simulink model "EKF_sim"  (R2021a)
settings: Solver=ode45  StartTime=0.0  StopTime=450  MaxStep=0.1  RelTol=1e-3  EnableMultiTasking=on
model workspace (MATLAB code in the model file + MAT data in the model file):
  L = 2.5
  v0 = 0
  xe0 = 0
  xn0 = 0
  theta0 = 0
  Ts = 1
  rr = [0 0 0 0 0 0 0 0 0 0 0 0 ... (9404 elements, 9404x1)]
  tt = [0 0.05 0.1 0.15 0.2 0.25 0.3 0.35 0.4 0.45 0.5 0.55 ... (9404 elements, 9404x1)]
  vv = [25 25 25 25 25 25 25 25 25 25 25 25 ... (9404 elements, 9404x1)]
libraries: simulink x2, pid_lib x2, sharedTrackingLibrary x1
(part 1 of 2)
settings Model: Creator=The MathWorks, Inc.  LastModifiedBy=angeloz
settings SolverCC: AlgebraicLoopSolver=TrustRegion
settings DataIOCC: SaveFormat=Array  SaveOutput=off  SignalLogging=off  DSMLogging=off  SaveTime=off  ReturnWorkspaceOutputs=off
settings OptimizationCC: LifeSpan=inf
settings DebuggingCC: AlgebraicLoopMsg=none  SolverPrmCheckMsg=warning  SFUnexpectedBacktrackingDiag=warning  SFNoUnconditionalDefaultTransitionDiag=warning  SFExecutionAtInitializationDiag=none  SFMachineParentedDataDiag=warning  ArithmeticOperatorsInVariantConditions=warning
settings HardwareCC: ProdBitPerPointer=32  ProdBitPerSizeT=32  ProdBitPerPtrDiffT=32  ProdLargestAtomicFloat=None  ProdIntDivRoundTo=Undefined  ProdEndianess=Unspecified  ProdWordSize=32  ProdHWDeviceType=32-bit Generic
settings ModelReferenceCC: PropagateSignalLabelsOutOfModel=off
settings SFSimCC: SimUseLocalCustomCode=off  CustomCodeUndefinedFunction=UseInterfaceOnly
settings RTWCC: RTWUseLocalCustomCode=off
settings CodeAppCC: StateflowObjectComments=on
settings GRTTargetCC: TargetLangStandard=C89/C90 (ANSI)
settings ConfigComp: CovMetricSettings=dw  CovSaveCumulativeToWorkspaceVar=on  CovSaveSingleToWorkspaceVar=on  CovExternalEMLEnable=off  CovSFcnEnable=off

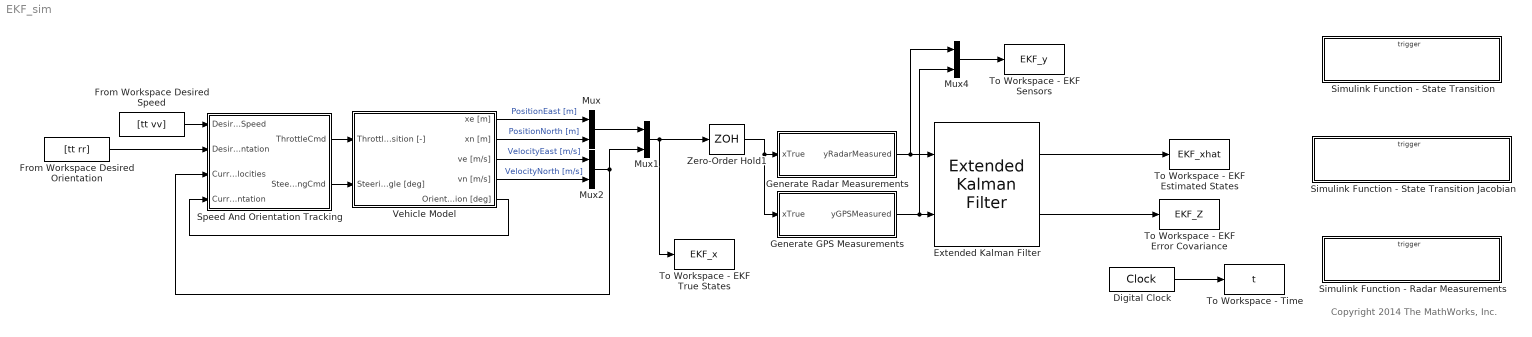
== system EKF_sim ==
  note: Copyright 2014 The MathWorks, Inc.
  Digital Clock : DigitalClock  SampleTime=Ts
  Extended Kalman Filter : sharedTrackingLibrary/Extended Kalman Filter  StateTransitionFcn=stateTransitionFcn  HasStateTransitionJacobianFcn=on  StateTransitionJacobianFcn=stateTransitionJacobianFcn  HasAdditiveProcessNoise=Nonadditive  ProcessNoise=[0.01 0; 0 0.01]  HasTimeVaryingProcessNoise=off  HasStateTransitionFcnExtraArgument=0  InitialState=[0; 0; 0; 0]  InitialStateCovariance=10  MeasurementFcn1=radarMeasurementFcn  HasMeasurementJacobianFcn1=off  HasMeasurementEnablePort1=off  HasAdditiveMeasurementNoise1=Nonadditive  MeasurementNoise1=[0.0025 0; 0 0.0025]  HasTimeVaryingMeasurementNoise1=off  HasMeasurementFcnExtraArgument1=0  MeasurementFcn2=gpsMeasurementFcn  HasMeasurementJacobianFcn2=off  HasMeasurementEnablePort2=off  HasAdditiveMeasurementNoise2=Additive  MeasurementNoise2=[100 0; 0 100]  HasTimeVaryingMeasurementNoise2=off  HasMeasurementFcnExtraArgument2=0  MeasurementFcn3=myMeasurementFcn  HasMeasurementJacobianFcn3=off  HasMeasurementEnablePort3=off  HasAdditiveMeasurementNoise3=Additive  MeasurementNoise3=1  HasTimeVaryingMeasurementNoise3=off  HasMeasurementFcnExtraArgument3=0  MeasurementFcn4=myMeasurementFcn  HasMeasurementJacobianFcn4=off  HasMeasurementEnablePort4=off  HasAdditiveMeasurementNoise4=Additive  MeasurementNoise4=1  HasTimeVaryingMeasurementNoise4=off  HasMeasurementFcnExtraArgument4=0  MeasurementFcn5=myMeasurementFcn  HasMeasurementJacobianFcn5=off  HasMeasurementEnablePort5=off  HasAdditiveMeasurementNoise5=Additive  MeasurementNoise5=1  HasTimeVaryingMeasurementNoise5=off  HasMeasurementFcnExtraArgument5=0  EnableMultirate=on  StateTransitionFcnSampleTime=0.05  MeasurementFcn1SampleTime=0.05  MeasurementFcn2SampleTime=1  MeasurementFcn3SampleTime=-1  MeasurementFcn4SampleTime=-1  MeasurementFcn5SampleTime=-1  UseCurrentEstimator=on  OutputStateCovariance=on  DataType=double  SampleTime=1  NumberOfMeasurements=2
      settings: SourceProductBaseCode=CT,DR,TF,ID,LP,NV,AR,RO,RR,UV,VE
  From Workspace Desired Orientation : FromWorkspace  VariableName=[tt rr]
  From Workspace Desired Speed : FromWorkspace  VariableName=[tt vv]
  Generate GPS Measurements : Subsystem
  Generate Radar Measurements : Subsystem
  Mux{,1..2,4} (4 alike) : Mux  Inputs=2
  Simulink Function - Radar Measurements : Subsystem  TreatAsAtomicUnit=on
  Simulink Function - State Transition : Subsystem  TreatAsAtomicUnit=on
  Simulink Function - State Transition Jacobian : Subsystem  TreatAsAtomicUnit=on
  Speed And Orientation Tracking : Subsystem
  To Workspace - EKF Error Covariance : ToWorkspace  VariableName=EKF_Z  SampleTime=-1
  To Workspace - EKF Estimated States : ToWorkspace  VariableName=EKF_xhat  SampleTime=-1
      settings: Save2DSignal=2-D array (concatenate along first dimension)
  To Workspace - EKF Sensors : ToWorkspace  VariableName=EKF_y  SampleTime=-1
      settings: Save2DSignal=2-D array (concatenate along first dimension)
  To Workspace - EKF True States : ToWorkspace  VariableName=EKF_x  SampleTime=Ts
      settings: Save2DSignal=2-D array (concatenate along first dimension)
  To Workspace - Time : ToWorkspace  VariableName=t  SampleTime=-1
      settings: Save2DSignal=2-D array (concatenate along first dimension)
  Vehicle Model : Subsystem
  Zero-Order Hold1 : ZeroOrderHold  SampleTime=Ts
  wires:
  Vehicle Model/2(xn [m]) -> Mux/2  "PositionNorth [m]"
  Vehicle Model/1(xe [m]) -> Mux/1  "PositionEast [m]"
  Digital Clock/1 -> To Workspace - Time/1
  Mux/1 -> Mux1/1
  Vehicle Model/4(vn [m/s]) -> Mux2/2  "VelocityNorth [m/s]"
  Vehicle Model/3(ve [m/s]) -> Mux2/1  "VelocityEast [m/s]"
  Mux2/1 -> Speed And Orientation Tracking/3(CurrentVelocities), Mux1/2
  Speed And Orientation Tracking/2(SteeringCmd) -> Vehicle Model/2("SteeringAngle [deg] ")
  Speed And Orientation Tracking/1(ThrottleCmd) -> Vehicle Model/1(ThrottlePosition [-])
  Vehicle Model/5(Orientation [deg]) -> Speed And Orientation Tracking/4(CurrentOrientation)
  From Workspace Desired Orientation/1 -> Speed And Orientation Tracking/2(DesiredOrientation)
  From Workspace Desired Speed/1 -> Speed And Orientation Tracking/1(DesiredSpeed)
  Extended Kalman Filter/1 -> To Workspace - EKF Estimated States/1
  Generate Radar Measurements/1(yRadarMeasured) -> Mux4/1, Extended Kalman Filter/1
  Generate GPS Measurements/1(yGPSMeasured) -> Mux4/2, Extended Kalman Filter/2
  Zero-Order Hold1/1 -> Generate GPS Measurements/1(xTrue), Generate Radar Measurements/1(xTrue)
  Mux4/1 -> To Workspace - EKF Sensors/1
  Extended Kalman Filter/2 -> To Workspace - EKF Error Covariance/1
  Mux1/1 -> To Workspace - EKF True States/1, Zero-Order Hold1/1
